simulink model "miniprojekt_nieliniowy"  (R2020a)
settings: Solver=ode15s  StartTime=0.0  StopTime=10.0  RelTol=1e-3
values from neighbouring files (symbols this model uses):
  c_p = 1000    [ch_stat.m]    (also in nieliniowy.m; nieliniowy_leveled.m; statespace_transmitancja.m; statespace_transmitancja_leveled.m)
  Cvp = c_p*ro_p*V_p    (= 180000)    [ch_stat.m]    (also in nieliniowy.m = 60000; nieliniowy_leveled.m = 60000; statespace_transmitancja.m = 60000; statespace_transmitancja_leveled.m = 60000)
  Cvw = c_p*ro_p*V_wew    (= 1080000)    [ch_stat.m]    (also in nieliniowy.m = 180000; nieliniowy_leveled.m = 180000; statespace_transmitancja.m = 180000; statespace_transmitancja_leveled.m = 180000)
  d_fp = 0    [nieliniowy.m]    (also in nieliniowy_leveled.m)
  d_qg = 0    [nieliniowy.m]    (also in nieliniowy_leveled.m; statespace_transmitancja.m; statespace_transmitancja_leveled.m)
  d_Tzew = 2    [nieliniowy.m]    (also in nieliniowy_leveled.m; statespace_transmitancja.m; statespace_transmitancja_leveled.m)
  fp1 = 0.5*fpN    (= 0.5)    [nieliniowy.m]    (also in nieliniowy_leveled.m; statespace_transmitancja.m = 2; statespace_transmitancja_leveled.m = 5)
  Kp = (c_p*ro_p*fpN*(TwewN-TpN))/(TpN-TzewN)    (= 54.5454545455)    [ch_stat.m]    (also in nieliniowy.m; nieliniowy_leveled.m; statespace_transmitancja.m; statespace_transmitancja_leveled.m)
  Kw = (qgN-c_p*ro_p*fpN*TwewN+c_p*ro_p*fpN*TpN)/(TwewN-TzewN)    (= 13.0434782609)    [ch_stat.m]    (also in nieliniowy.m; nieliniowy_leveled.m; statespace_transmitancja.m; statespace_transmitancja_leveled.m)
  qg1 = 0.5*qgN    (= 750)    [nieliniowy.m]    (also in nieliniowy_leveled.m; statespace_transmitancja.m; statespace_transmitancja_leveled.m)
  ro_p = 1.2    [ch_stat.m]    (also in nieliniowy.m; nieliniowy_leveled.m; statespace_transmitancja.m; statespace_transmitancja_leveled.m)
  Tp0 = (c_p*ro_p*fp1*qg1)/(c_p*ro_p*fp1*(Kp+Kw)+Kw*Kp)+Tzew1    (= 13.9051724138)    [nieliniowy.m]    (also in nieliniowy_leveled.m; statespace_transmitancja.m = 14.0480349345; statespace_transmitancja_leveled.m = 14.0770577933)
  Twew0 = (c_p*ro_p*fp1*Tp0+Kp*Tp0-Kp*Tzew1)/(c_p*ro_p*fp1)    (= 14.8965517241)    [nieliniowy.m]    (also in nieliniowy_leveled.m; statespace_transmitancja.m = 14.2991266376; statespace_transmitancja_leveled.m = 14.1777583187)
  Tzew1 = TzewN+5    (= 3)    [nieliniowy.m]    (also in nieliniowy_leveled.m; statespace_transmitancja.m; statespace_transmitancja_leveled.m)
settings Model: Creator=Jakub Szymkowiak  LastModifiedBy=Jakub Szymkowiak

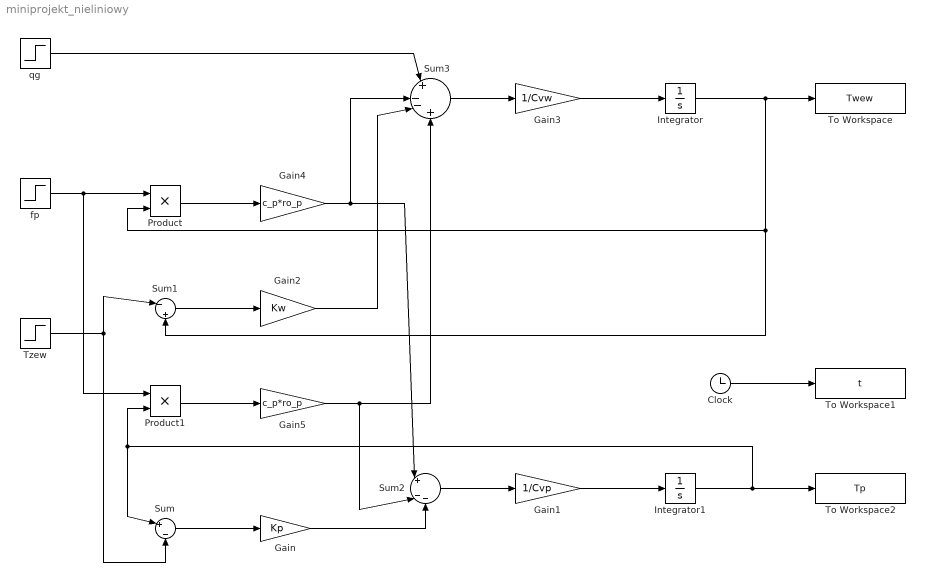
== system miniprojekt_nieliniowy ==
  Clock : Clock
  Gain : Gain  Gain=Kp
  Gain1 : Gain  Gain=1/Cvp
  Gain2 : Gain  Gain=Kw
  Gain3 : Gain  Gain=1/Cvw
  Gain4 : Gain  Gain=c_p*ro_p
  Gain5 : Gain  Gain=c_p*ro_p
  Integrator : Integrator  InitialCondition=Twew0
  Integrator1 : Integrator  InitialCondition=Tp0
  Product : Product
  Product1 : Product
  Sum : Sum  Inputs=|+|-
  Sum1 : Sum  Inputs=|-|+
  Sum2 : Sum  Inputs=|+|--
  Sum3 : Sum  Inputs=|+|--|+
  To Workspace : ToWorkspace  VariableName=Twew  SaveFormat=Timeseries  SampleTime=-1
  To Workspace1 : ToWorkspace  VariableName=t  SaveFormat=Timeseries  SampleTime=-1
  To Workspace2 : ToWorkspace  VariableName=Tp  SaveFormat=Timeseries  SampleTime=-1
  Tzew : Step  Before=Tzew1  After=Tzew1+d_Tzew  SampleTime=0
  fp : Step  Before=fp1  After=fp1+d_fp  SampleTime=0
  qg : Step  Before=qg1  After=qg1 + d_qg  SampleTime=0
  wires:
  Clock/1 -> To Workspace1/1
  qg/1 -> Sum3/1
  fp/1 -> Product1/1, Product/1
  Product/1 -> Gain4/1
  Sum3/1 -> Gain3/1
  Gain3/1 -> Integrator/1
  Integrator/1 -> Sum1/2, Product/2, To Workspace/1
  Tzew/1 -> Sum/2, Sum1/1
  Product1/1 -> Gain5/1
  Sum1/1 -> Gain2/1
  Sum/1 -> Gain/1
  Gain/1 -> Sum2/3
  Sum2/1 -> Gain1/1
  Gain1/1 -> Integrator1/1
  Integrator1/1 -> Sum/1, Product1/2, To Workspace2/1
  Gain4/1 -> Sum2/1, Sum3/2
  Gain5/1 -> Sum2/2, Sum3/4
  Gain2/1 -> Sum3/3
